simulink model "exercise2_model"  (R2015a)
settings: Solver=ode45  StartTime=0.0  StopTime=10.0  RelTol=1e-3
values from neighbouring files (symbols this model uses):
  c1 = 5    [exercise2.m]
  c2 = 10    [exercise2.m]
  den = [1 1/R*C 1/L*C]    [exercise1.m]    (also in exercise2.m = [1 1 (1/(R*C) + 2*qp*C)]; exercise3.m = [1 2*Ws_d*zeta_d Ws_d^2])
  E = 30    [exercise2.m]
  num = [1 0 1/L*C]    [exercise1.m]    (also in exercise2.m = [1/(R*C*L)]; exercise3.m = [gain_d*(Ws_d^2)])
  R = 5    [exercise1.m]    (also in exercise2.m = 50)
  u0 = 80    [exercise2.m]
settings Model: Creator=Estudiantes  LastModifiedBy=Daniel Santos
settings DataIOCC: SignalLoggingSaveFormat=ModelDataLogs
settings OptimizationCC: ExpressionDepthLimit=2147483647
settings DebuggingCC: UnderspecifiedInitializationDetection=Classic  MergeDetectMultiDrivingBlocksExec=none  SolverPrmCheckMsg=warning  FcnCallInpInsideContextMsg=EnableAllAsWarning  StateNameClashWarn=warning

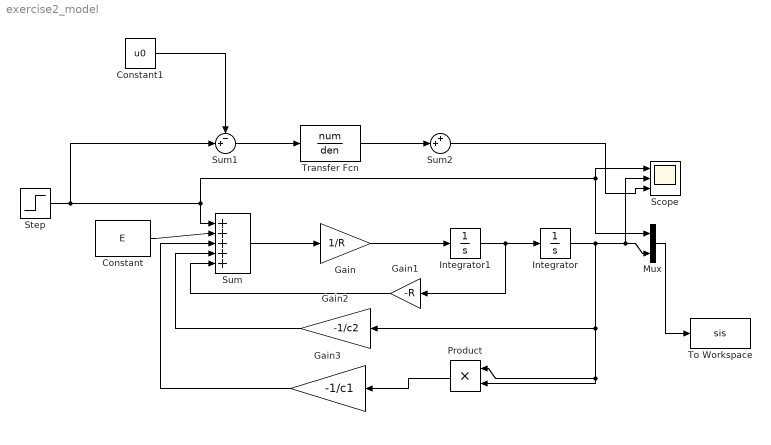
== system exercise2_model ==
  Constant : Constant  Value=E
  Constant1 : Constant  Value=u0
  Gain : Gain  Gain=1/R
  Gain1 : Gain  Gain=-R
  Gain2 : Gain  Gain=-1/c2
  Gain3 : Gain  Gain=-1/c1
  Integrator : Integrator
  Integrator1 : Integrator
  Mux : Mux  Inputs=2
  Product : Product  RndMeth=Zero
  Scope : Scope  NumInputPorts=3
      settings: ShowLegends=on  YMin=-5~-5~-5  YMax=5~5~5
  Step : Step  After=-1  SampleTime=0
  Sum : Sum  Inputs=|+++++
  Sum1 : Sum  Inputs=-+|
  Sum2 : Sum  Inputs=++|
  To Workspace : ToWorkspace  VariableName=sis  SaveFormat=Structure With Time  SampleTime=-1
  Transfer Fcn : TransferFcn  Numerator=num  Denominator=den
  wires:
  Integrator/1 -> Product/1, Product/2, Gain2/1, Mux/2, Scope/2
  Integrator1/1 -> Integrator/1, Gain1/1
  Gain/1 -> Integrator1/1
  Sum/1 -> Gain/1
  Gain1/1 -> Sum/5
  Product/1 -> Gain3/1
  Gain2/1 -> Sum/4
  Gain3/1 -> Sum/3
  Mux/1 -> To Workspace/1
  Constant/1 -> Sum/2
  Step/1 -> Sum/1, Mux/1, Scope/1, Sum1/2
  Sum1/1 -> Transfer Fcn/1
  Transfer Fcn/1 -> Sum2/2
  Sum2/1 -> Scope/3
  Constant1/1 -> Sum1/1
